simulink library "ME598_ProjectLibrary"  (R2024a)
settings: Solver=ode23t  StartTime=0.0  StopTime=10.0  RelTol=1e-3
InitFcn:
  | RPInit
libraries: RoboticsPlayground x9, RP_Simulator_Components x6, robotmobilelib x1
settings Model: Creator=Mishah  LastModifiedBy=sathyaprasadreddypatlolla
settings SolverCC: AlgebraicLoopSolver=TrustRegion
settings DebuggingCC: UnconnectedInputMsg=warning  UnconnectedOutputMsg=warning  UnconnectedLineMsg=warning
settings ModelReferenceCC: EnableRefExpFcnMdlSchedulingChecks=on
settings RTWCC: GPUComputeCapability=3.5  DLArmComputeVersion=19.05

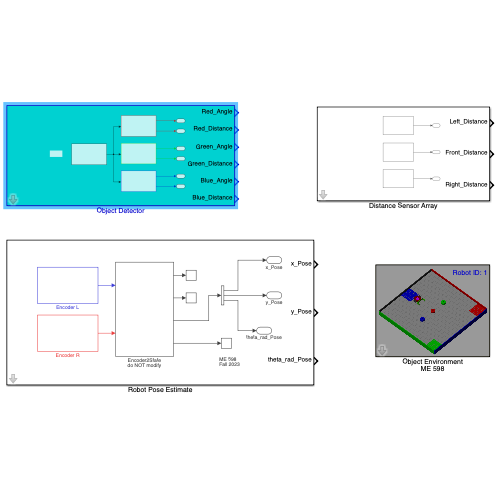
[thumbnail: Simulink's stored preview of the top-level diagram]
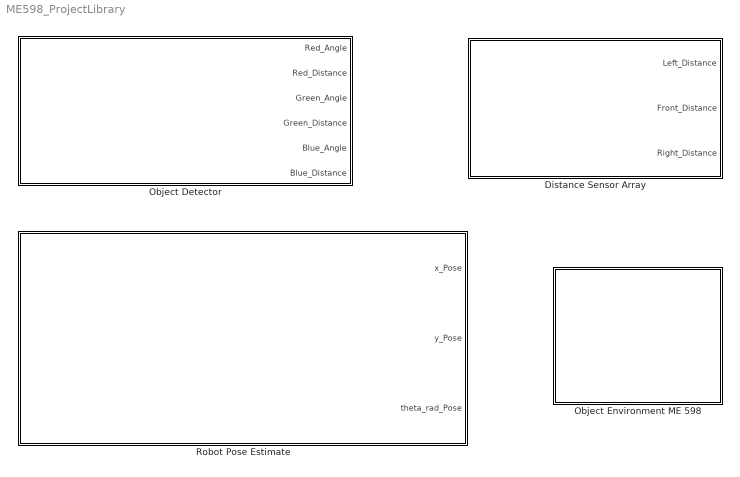
== system ME598_ProjectLibrary ==
  Distance Sensor Array : Subsystem  mask(Distance Sensor Array){}
      mask help:
      | Custom distance sensor array block based on the Robotics Playground library blocks.
      |
      | Right click and navigate to Mask --> Look Under Mask to inspect configuration parameters for the blocks within this subsystem.
      |
      | Each internal block's settings are purposefully locked to predetermined values to avoid unintentional changes.
  Object Detector : Subsystem  mask(Object Detector){}
      mask help:
      | Custom object detection block based on the Robotics Playground library blocks.
      |
      | Right click and navigate to Mask --> Look Under Mask to inspect configuration parameters for the blocks within this subsystem.
      |
      | Each internal block's settings are purposefully locked to predetermined values to avoid unintentional changes.
  Object Environment ME 598 : Subsystem  mask(RP Object Environment){obj1=on, objPose1=[0 1.5], objColor1=Red, obj2=off, objPose2=[0 0], objColor2=Green, obj3=on, objPose3=[0 -1.5], objColor3=Blue, obj4=off, objPose4=[-0.61298      2.9263], objColor4=Red, obj5=off, objPose5=[-0.61298      2.9263], objColor5=Red, arenaLength=5, arenaWidth=5, robotId=1, wheelBase=0.5, wheelRadius=0.1, robotColor=[0.5 0 0], startPose=[-1.5 0]}
      mask prompts: obj1 "Enabled"; objPose1 "Initial position X Y [m]"; objColor1 "Color"; obj2 "Enabled"; objPose2 "Initial position X Y [m]"; objColor2 "Color"; obj3 "Enabled"; objPose3 "Initial position X Y [m]"; objColor3 "Color"; obj4 "Enabled"; objPose4 "Initial position X Y [m]"; objColor4 "Color"; obj5 "Enabled"; objPose5 "Initial position X Y [m]"; objColor5 "Color"; arenaLength "Length [m]"; arenaWidth "Width [m]"; robotId "Robot ID"; wheelBase "Distance between wheels [m]"; wheelRadius "Wheel radius [m]"; robotColor "Color [R G B]"; startPose "Initial Position X Y [m]"
      mask help:
      | This block has been customized and tested with MATLAB R2023a and Robotics Playground v23.1.1.0
      | for Stevens Institute of Technology course ME 598, Fall 2023.
      |
      | It contains a virtual environment for a single robot to interact with walls and moveable objects. For your course project, only the sensors and actuators provided in the file ** Project_start.slx ** may be used for sensing and to actuate the robot.
      |
      | Motor mapping for the robot is as follows:
      |
      | Motor 1 -> Left wheel motor **torque**
      | Motor 2 -> Right wheel motor **torque**
      settings: CopyFcn=|
      | set_param(gcs,'InitFcn','RPInit');
      | set_param(gcs,'Solver','ode23t');
      | set_param(gcs, 'EnablePacing', 'on')
      | set_param(gcs, 'PacingRate', 1)
      mask Help: web('object_arena.htm')
      mask Callback obj1: setObjects(gcb)
      mask Callback objPose1: setObjects(gcb)
      mask TypeOptions objColor1: Red | Green | Blue
      mask Callback objColor1: setObjects(gcb)
      mask Callback obj2: setObjects(gcb)
      mask Callback objPose2: setObjects(gcb)
      mask TypeOptions objColor2: Red | Green | Blue
      mask Callback objColor2: setObjects(gcb)
      mask Callback obj3: setObjects(gcb)
      mask Callback objPose3: setObjects(gcb)
      mask TypeOptions objColor3: Red | Green | Blue
      mask Callback objColor3: setObjects(gcb)
      mask Callback obj4: setObjects(gcb)
      mask Callback objPose4: setObjects(gcb)
      mask TypeOptions objColor4: Red | Green | Blue
      mask Callback objColor4: setObjects(gcb)
      mask Callback obj5: setObjects(gcb)
      mask Callback objPose5: setObjects(gcb)
      mask TypeOptions objColor5: Red | Green | Blue
      mask Callback objColor5: setObjects(gcb)
      mask DialogControl objT Prompt: Object settings
      mask DialogControl objc1 Prompt: Left Object
      mask DialogControl objc2 Prompt: Center Object
      mask DialogControl objc3 Prompt: Right Object
      mask DialogControl objc4 Prompt: Object 4
      mask DialogControl objc5 Prompt: Object 5
      mask DialogControl Container6 Prompt: Arena settings
      mask DialogControl Container4 Prompt: Robot settings
      mask Display:
      | color('white');
      | plot([100,100,100,100]*1,[100,100,100,100]*1);
      | plot([100,100,100,100]*0,[100,100,100,100]*0);
      | image('ObjectEnv.PNG')
      | color('blue');
      | id=eval(get_param(gcb,'robotId'));
      | text(99, 92, ['Robot ID: ' num2str(id)], 'horizontalAlignment', 'right');
  Robot Pose Estimate : Subsystem  mask(Robot Pose Estimate){}
      mask help:
      | Custom robot pose estimate block based on the Robotics Playground library blocks. Outputs are x, y, and theta (radian) estimates of the robot's instantaneous pose as determined from encoder values and the robot's differential drive kinematics.
      |
      | Right click and navigate to Mask --> Look Under Mask to inspect configuration parameters for the blocks within this subsystem.
      |
      | Each internal block's settings are purposefully locked to predetermined values to avoid unintentional changes.

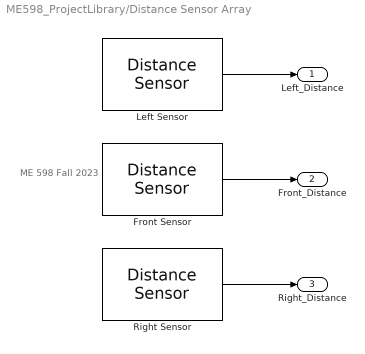
== system ME598_ProjectLibrary/Distance Sensor Array ==
  note: ME 598
      | Fall 2023
  Front Sensor : RoboticsPlayground/Basic Sensors and Actuators/Distance Sensor  robotId=1  maxSenRange=2  minSenRange=0.02  senRes=0.01  sensOff=[0.25 0]  sensOffDeg=0  sensorTs=0.1
      settings: SourceProductName=Robotics Playground
  Left Sensor : RoboticsPlayground/Basic Sensors and Actuators/Distance Sensor  robotId=1  maxSenRange=2  minSenRange=0.02  senRes=0.01  sensOff=[0.15 0.15]  sensOffDeg=90  sensorTs=0.1
      settings: SourceProductName=Robotics Playground
  Right Sensor : RoboticsPlayground/Basic Sensors and Actuators/Distance Sensor  robotId=1  maxSenRange=2  minSenRange=0.02  senRes=0.01  sensOff=[0.15 -0.15]  sensOffDeg=-90  sensorTs=0.1
      settings: SourceProductName=Robotics Playground
  Left_Distance : Outport
  Front_Distance : Outport  Port=2
  Right_Distance : Outport  Port=3
  wires:
  Front Sensor/1 -> Front_Distance/1
  Left Sensor/1 -> Left_Distance/1
  Right Sensor/1 -> Right_Distance/1

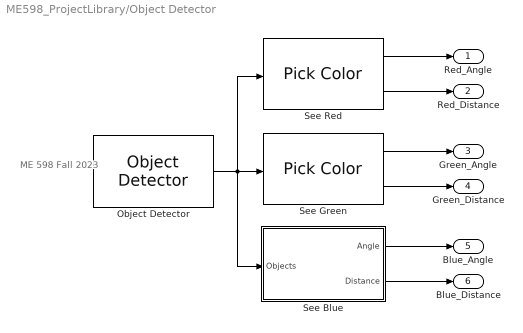
== system ME598_ProjectLibrary/Object Detector ==
  note: ME 598
      | Fall 2023
  Object Detector : RoboticsPlayground/Advanced Sensors/Object Detector  robotId=1  maxSenRange=2  sensFOV=60  sensOff=[0 0]  sensOffDeg=0  sensorTs=0.1
      settings: SourceProductName=Robotics Playground
  See Blue : Subsystem  mask(RP Pick Color){colorSelection=Blue}
      mask prompts: colorSelection "Color"
      mask help: This block receives all the detections from the output of a RP Object Detector and outputs the angle in degrees and distance in meters to the nearest object of the selected color.
      mask init:
      | colorSelection=get_param(gcb,'colorSelection');
      | 
      | if strcmp(colorSelection,'Red')
      |     color=1;
      | elseif strcmp(colorSelection,'Green')
      |     color=2;
      | else
      |     color=3;
      | end
      mask Help: web('pick_color.htm')
      mask TypeOptions colorSelection: Red | Green | Blue
      mask Display:
      | colorSelection=get_param(gcb,'colorSelection');
      | 
      | if strcmp(colorSelection,'Red')
      |     image('RedObjD.png','center')
      | elseif strcmp(colorSelection,'Green')
      |     image('GreenObjD.png','center')
      | else
      |     image('BlueObjD.png','center')
      | end
      | 
      | color('black');
      | port_label('input', 1', 'Objects');
      | port_label('output', 1', 'Angle');
      | port_label('output', 2', 'Distance');
  See Green : RoboticsPlayground/Advanced Sensors/Pick Color  colorSelection=Green
      settings: SourceProductName=Robotics Playground
  See Red : RoboticsPlayground/Advanced Sensors/Pick Color  colorSelection=Red
      settings: SourceProductName=Robotics Playground
  Red_Angle : Outport
  Red_Distance : Outport  Port=2
  Green_Angle : Outport  Port=3
  Green_Distance : Outport  Port=4
  Blue_Angle : Outport  Port=5
  Blue_Distance : Outport  Port=6
  wires:
  See Green/2 -> Green_Distance/1
  See Green/1 -> Green_Angle/1
  See Blue/2(Distance) -> Blue_Distance/1
  See Red/1 -> Red_Angle/1
  See Blue/1(Angle) -> Blue_Angle/1
  Object Detector/1 -> See Blue/1(Objects), See Green/1, See Red/1
  See Red/2 -> Red_Distance/1

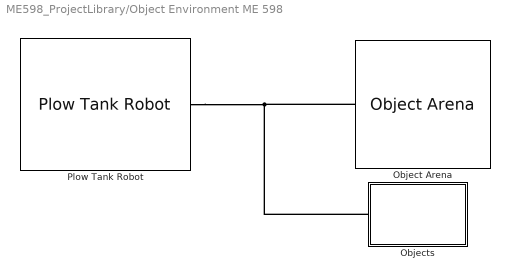
== system ME598_ProjectLibrary/Object Environment ME 598 ==
  Object Arena : RP_Simulator_Components/Object Arena  length=arenaLength  width=arenaWidth  robotRadius=wheelBase/2
  Objects : Subsystem
  Plow Tank Robot : RoboticsPlayground/Environments/Object Environment/Plow Tank Robot  robotId=robotId  wheelRadius=wheelRadius  wheelBase=wheelBase  wheelThickness=0.025  chassisThickness=0.05  startPose=startPose  choice=off  sensorTs=0.05  wheelMass=0.2  chassisMass=0.5  maxWheelTorque=1  floorSize=[arenaLength arenaWidth]  wheelColor=[0.25 0.25 0.25]  chassisColor=robotColor
      settings: SourceProductName=Robotics Playground
  connections:
  Objects/LConn1 -- Plow Tank Robot/RConn1 -- Object Arena/LConn1

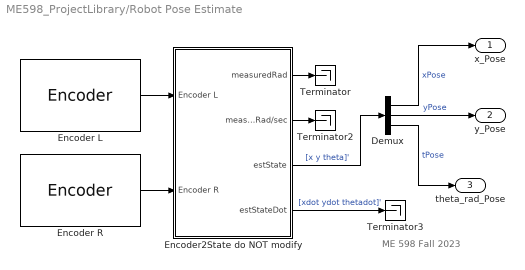
== system ME598_ProjectLibrary/Robot Pose Estimate ==
  note: ME 598
      | Fall 2023
  Demux : Demux  Outputs=3
  Encoder L : RoboticsPlayground/Basic Sensors and Actuators/Encoder  robotId=1  motorChoice=1  rstChoice=No reset  ticks=180  detectDir=on  sensorTs=0.1
      settings: SourceProductName=Robotics Playground
  Encoder R : RoboticsPlayground/Basic Sensors and Actuators/Encoder  robotId=1  motorChoice=2  rstChoice=No reset  ticks=180  detectDir=on  sensorTs=0.1
      settings: SourceProductName=Robotics Playground
  Encoder2State do NOT modify : Subsystem
  Terminator : Terminator
  Terminator2 : Terminator
  Terminator3 : Terminator
  x_Pose : Outport
  y_Pose : Outport  Port=2
  theta_rad_Pose : Outport  Port=3
  wires:
  Encoder2State do NOT modify/4(estStateDot) -> Terminator3/1  "[xdot ydot thetadot]'"
  Encoder L/1 -> Encoder2State do NOT modify/1(Encoder L)
  Encoder2State do NOT modify/2(measuredRad/sec) -> Terminator2/1
  Demux/2 -> y_Pose/1  "yPose"
  Encoder R/1 -> Encoder2State do NOT modify/2(Encoder R)
  Demux/1 -> x_Pose/1  "xPose"
  Demux/3 -> theta_rad_Pose/1  "tPose"
  Encoder2State do NOT modify/3(estState) -> Demux/1  "[x y theta]'"
  Encoder2State do NOT modify/1(measuredRad) -> Terminator/1

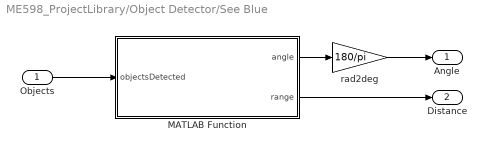
== system ME598_ProjectLibrary/Object Detector/See Blue ==
  Objects : Inport
  MATLAB Function : MATLAB Function  TreatAsAtomicUnit=on
  rad2deg : Gain  Gain=180/pi
  Angle : Outport  VectorParamsAs1DForOutWhenUnconnected=off
  Distance : Outport  Port=2  VectorParamsAs1DForOutWhenUnconnected=off
  wires:
  Objects/1 -> MATLAB Function/1(objectsDetected)
  MATLAB Function/1(angle) -> rad2deg/1
  MATLAB Function/2(range) -> Distance/1
  rad2deg/1 -> Angle/1

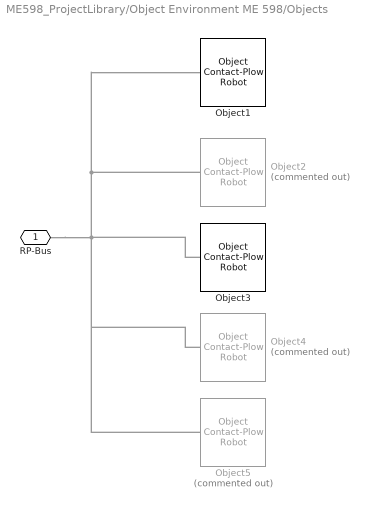
== system ME598_ProjectLibrary/Object Environment ME 598/Objects ==
  Object1 : RP_Simulator_Components/Object Contact-Plow Robot  objectId=1  Pose=[0 1.5]  objRadius=0.15  robotRadius=0.25  height=0.2  color=[0.8 0 0]  length=arenaLength  width=arenaWidth
  Object2 : RP_Simulator_Components/Object Contact-Plow Robot  Commented=on  objectId=2  Pose=[0 0]  objRadius=0.15  robotRadius=0.25  height=0.2  color=[0 0.8 0]  length=arenaLength  width=arenaWidth
  Object3 : RP_Simulator_Components/Object Contact-Plow Robot  objectId=3  Pose=[0 -1.5]  objRadius=0.15  robotRadius=0.25  height=0.2  color=[0 0 0.8]  length=arenaLength  width=arenaWidth
  Object4 : RP_Simulator_Components/Object Contact-Plow Robot  Commented=on  objectId=4  Pose="[-0.61298      2.9263]"  objRadius=0.15  robotRadius=0.25  height=0.2  color=[0.8 0 0]  length=arenaLength  width=arenaWidth
  Object5 : RP_Simulator_Components/Object Contact-Plow Robot  Commented=on  objectId=5  Pose="[-0.61298      2.9263]"  objRadius=0.15  robotRadius=0.25  height=0.2  color=[0.8 0 0]  length=arenaLength  width=arenaWidth
  RP-Bus : PMIOPort  Side=Left
  connections:
  Object2/LConn1 -- RP-Bus/RConn1 -- Object4/LConn1 -- Object5/LConn1 -- Object3/LConn1 -- Object1/LConn1

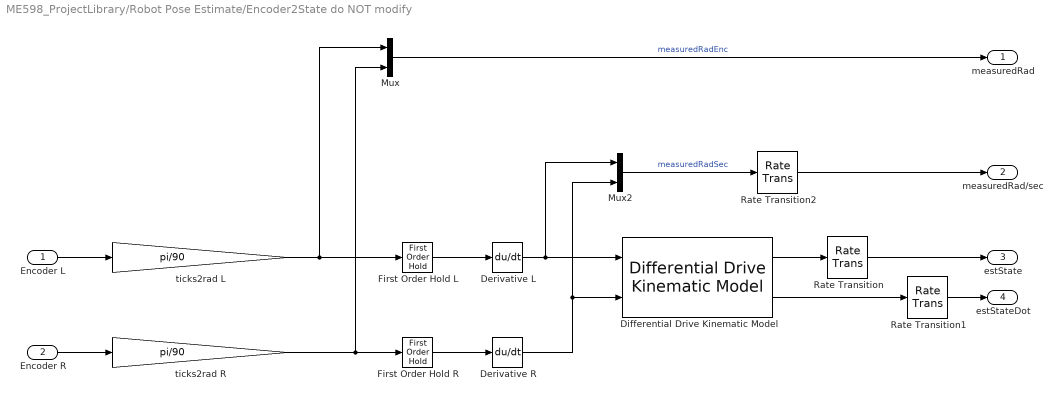
== system ME598_ProjectLibrary/Robot Pose Estimate/Encoder2State do NOT modify ==
  Encoder L : Inport
  Encoder R : Inport  Port=2
  Derivative L : Derivative
  Derivative R : Derivative
  Differential Drive Kinematic Model : robotmobilelib/Differential Drive Kinematic Model  VehicleInputs=Wheel Speeds  WheelRadius=0.1  WheelSpeedRange=[-inf inf]  TrackWidth=0.5  InitialState=[-1.5; 0; 0]  SimulateUsing=Interpreted execution
  First Order Hold L : FirstOrderHold  ErrorTolerance=inf
  First Order Hold R : FirstOrderHold  ErrorTolerance=inf
  Mux : Mux  Inputs=2
  Mux2 : Mux  Inputs=2
  Rate Transition : RateTransition  OutPortSampleTime=0.1
  Rate Transition1 : RateTransition  OutPortSampleTime=0.1
  Rate Transition2 : RateTransition  OutPortSampleTime=0.1
  ticks2rad L : Gain  Gain=pi/90
  ticks2rad R : Gain  Gain=pi/90
  measuredRad : Outport
  measuredRad/sec : Outport  Port=2
  estState : Outport  Port=3
  estStateDot : Outport  Port=4
  wires:
  Rate Transition2/1 -> measuredRad/sec/1
  Rate Transition1/1 -> estStateDot/1
  Rate Transition/1 -> estState/1
  Encoder L/1 -> ticks2rad L/1
  Differential Drive Kinematic Model/2 -> Rate Transition1/1
  ticks2rad L/1 -> First Order Hold L/1, Mux/1
  Mux/1 -> measuredRad/1  "measuredRadEnc"
  First Order Hold L/1 -> Derivative L/1
  Encoder R/1 -> ticks2rad R/1
  First Order Hold R/1 -> Derivative R/1
  Derivative L/1 -> Differential Drive Kinematic Model/1, Mux2/1
  Mux2/1 -> Rate Transition2/1  "measuredRadSec"
  Derivative R/1 -> Differential Drive Kinematic Model/2, Mux2/2
  ticks2rad R/1 -> First Order Hold R/1, Mux/2
  Differential Drive Kinematic Model/1 -> Rate Transition/1

== matlab function ME598_ProjectLibrary/Object Detector/See Blue/MATLAB Function ==
  data: objectsDetected input size=[5 3]; angle output; range output; color parameter
function [angle,range] = pickColor(objectsDetected, color)
%#codegen

if ~isempty(objectsDetected)
    colorDetections=objectsDetected(:,3)==color;
    if any(colorDetections)
        colorObjects=objectsDetected(colorDetections,1:2);
        angle=colorObjects(1,2);
        range=colorObjects(1,1);
    else
        angle=NaN;
        range=NaN;
    end
else
    angle=NaN;
    range=NaN;
end
